simulink model "RoboPies"  (R2025b)
settings: Solver=ode23t  StartTime=0.0  StopTime=Tf  RelTol=1e-2  AbsTol=1e-2  EnableMultiTasking=on
values from neighbouring files (symbols this model uses):
  k = 2    [init_PID.m]
  x = 0.25    [init_PID.m]
undefined symbols (not defined in the file or in its folder): bias, foot_radius, ground_offset, hip_max_angle, hip_min_angle, initial_hip_angle, initial_knee_angle, knee_max_angle, knee_min_angle, lower_leg, max_a, max_friction_force, max_hip_speed, max_knee_speed, max_magnitude_force, max_torque, max_v, torso, upper_leg, X, Y, Z
libraries: nesl_utility x44, sm_lib x36, rllib x1
(part 1 of 2)
settings Model: Creator=filip  LastModifiedBy=filip
settings SolverCC: ZeroCrossAlgorithm=Adaptive  MaxZcPerStep=1.0
settings DataIOCC: LimitDataPoints=on  MaxDataPoints=10000
settings OptimizationCC: ReuseModelBlockBuffer=off  LifeSpan=inf
settings DebuggingCC: AlgebraicLoopMsg=none  UnconnectedInputMsg=warning  UnconnectedOutputMsg=warning  UnconnectedLineMsg=warning  AllowSymbolicDim=off  SubsystemReferenceDiagnosticForUnitTest=warning  SFUnexpectedBacktrackingDiag=warning  SFNoUnconditionalDefaultTransitionDiag=warning  SFExecutionAtInitializationDiag=none  ArithmeticOperatorsInVariantConditions=warning
settings ModelReferenceCC: EnableRefExpFcnMdlSchedulingChecks=on
settings SFSimCC: SimUseLocalCustomCode=off  CustomCodeUndefinedFunction=UseInterfaceOnly
settings RTWCC: RTWUseLocalCustomCode=off  GPUComputeCapability=3.5  DLArmComputeVersion=19.05
settings CodeAppCC: StateflowObjectComments=on
settings GRTTargetCC: TargetLangStandard=C89/C90 (ANSI)
settings ConfigComp: CovMetricSettings=dw  CovSaveCumulativeToWorkspaceVar=on  CovSaveSingleToWorkspaceVar=on  CovExternalEMLEnable=off  CovSFcnEnable=off
settings SimscapeCC: SimscapeLogType=all  SimscapeLogSimulationStatistics=on  SimscapeLogDataHistory=10000.0

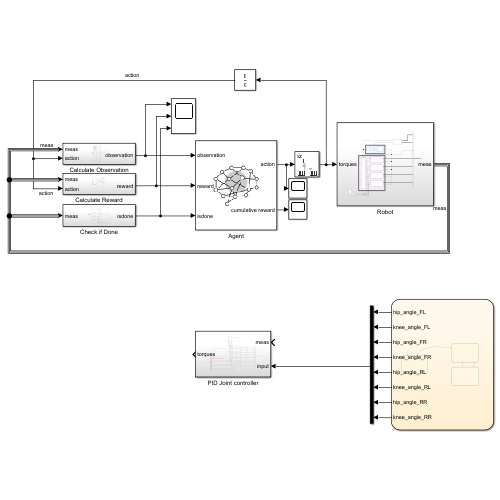
[thumbnail: Simulink's stored preview of the top-level diagram]
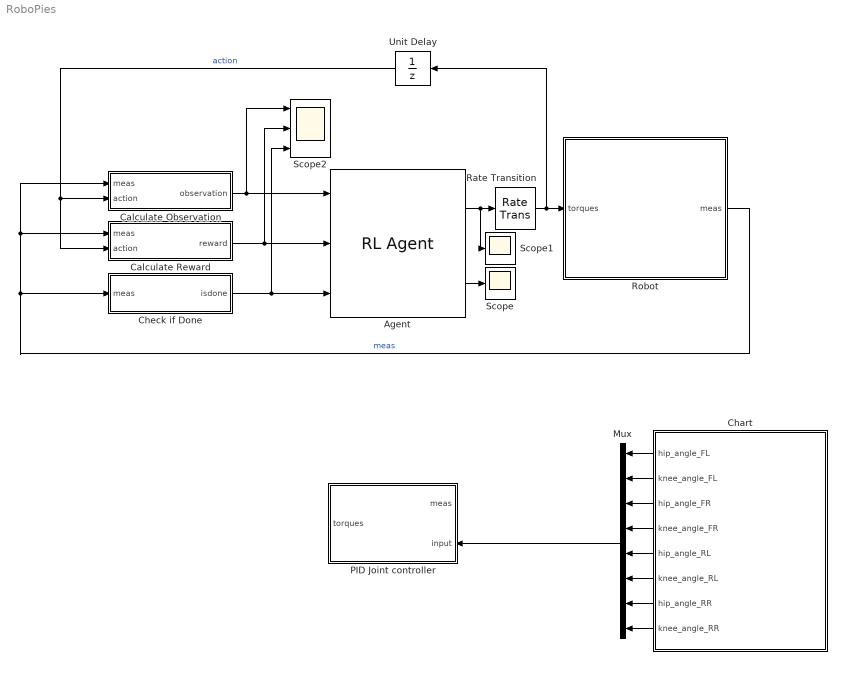
== system RoboPies ==
  Agent : rllib/RL Agent  Agent=agent  ExternalActionAsInput=off  ProvideLastAction=off  ProvideCumRwd=on  TreatAsDirectFeedthrough=on  UseStrictObservationDataTypes=off
  Calculate Observation : Subsystem
  Calculate Reward : Subsystem
  Chart : Stateflow chart  TreatAsAtomicUnit=on
  Check if Done : Subsystem
  Mux : Mux  Inputs=8
  PID Joint controller : Subsystem
  Rate Transition : RateTransition
  Robot : Subsystem
  Scope : Scope
  Scope1 : Scope
      settings: ActiveDisplayYMinimum=-2.81408298770246  ActiveDisplayYMaximum=3.6973431282332014  DataLoggingVariableName=ScopeData2
  Scope2 : Scope  NumInputPorts=3
      settings: ActiveDisplayYMinimum=-11.968223752166544  ActiveDisplayYMaximum=10.451088168830223  DataLoggingVariableName=ScopeData4
  Unit Delay : UnitDelay  SampleTime=-1  HasFrameUpgradeWarning=on
  wires:
  Chart/3(hip_angle_FR) -> Mux/3
  Chart/5(hip_angle_RL) -> Mux/5
  Chart/7(hip_angle_RR) -> Mux/7
  Chart/1(hip_angle_FL) -> Mux/1
  Chart/6(knee_angle_RL) -> Mux/6
  Chart/2(knee_angle_FL) -> Mux/2
  Chart/4(knee_angle_FR) -> Mux/4
  Chart/8(knee_angle_RR) -> Mux/8
  Mux/1 -> PID Joint controller/2(input)
  Calculate Reward/1(reward) -> Scope2/2, Agent/2
  Calculate Observation/1(observation) -> Scope2/1, Agent/1
  Robot/1(meas) -> Calculate Observation/1(meas), Calculate Reward/1(meas), Check if Done/1(meas)  "meas"
  Unit Delay/1 -> Calculate Reward/2(action), Calculate Observation/2(action)  "action"
  Check if Done/1(isdone) -> Scope2/3, Agent/3
  Agent/2 -> Scope/1
  Agent/1 -> Rate Transition/1, Scope1/1
  Rate Transition/1 -> Robot/1(torques), Unit Delay/1

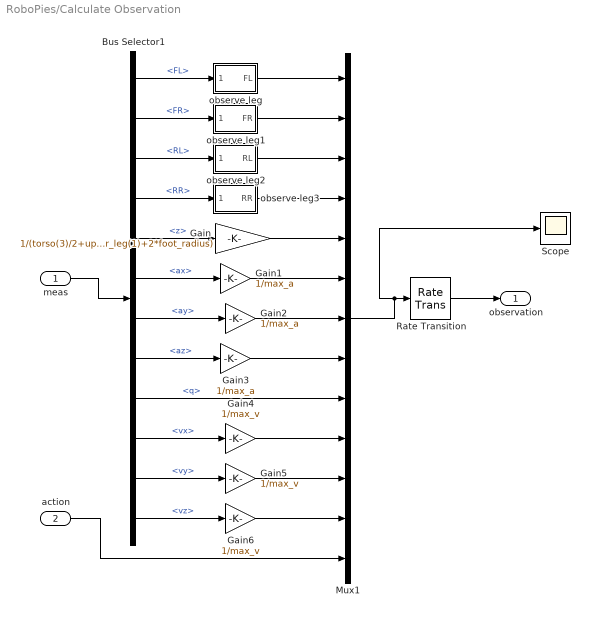
== system RoboPies/Calculate Observation ==
  meas : Inport
  action : Inport  Port=2
  Bus Selector1 : BusSelector  OutputSignals=FL,FR,RL,RR,translation.z,translation.ax,translation.ay,translation.az,rotation.q,translation.vx,translation.vy,translation.vz
  Gain : Gain  Gain=1/(torso(3)/2+upper_leg(1)+lower_leg(1)+2*foot_radius)
  Gain1 : Gain  Gain=1/max_a
  Gain2 : Gain  Gain=1/max_a
  Gain3 : Gain  Gain=1/max_a
  Gain4 : Gain  Gain=1/max_v
  Gain5 : Gain  Gain=1/max_v
  Gain6 : Gain  Gain=1/max_v
  Mux1 : Mux  Inputs=13
  Rate Transition : RateTransition  OutPortSampleTime=T
  Scope : Scope
      settings: ActiveDisplayYMinimum=-5.1137479560715171  ActiveDisplayYMaximum=2.9584463962824925  DataLoggingVariableName=ScopeData10
  observe leg : Subsystem
  observe leg1 : Subsystem
  observe leg2 : Subsystem
  observe leg3 : Subsystem
  observation : Outport
  wires:
  meas/1 -> Bus Selector1/1
  Rate Transition/1 -> observation/1
  Mux1/1 -> Scope/1, Rate Transition/1
  Bus Selector1/1 -> observe leg/1(<FL>)  "<FL>"
  Bus Selector1/2 -> observe leg1/1(<FR>)  "<FR>"
  Bus Selector1/3 -> observe leg2/1(<RL>)  "<RL>"
  Bus Selector1/4 -> observe leg3/1(<RR>)  "<RR>"
  observe leg3/1(RR) -> Mux1/4
  observe leg2/1(RL) -> Mux1/3
  observe leg1/1(FR) -> Mux1/2
  Bus Selector1/5 -> Gain/1  "<z>"
  Gain/1 -> Mux1/5
  Bus Selector1/6 -> Gain1/1  "<ax>"
  Bus Selector1/8 -> Gain3/1  "<az>"
  Bus Selector1/7 -> Gain2/1  "<ay>"
  Gain1/1 -> Mux1/6
  Gain2/1 -> Mux1/7
  Gain3/1 -> Mux1/8
  observe leg/1(FL) -> Mux1/1
  Bus Selector1/9 -> Mux1/9  "<q>"
  action/1 -> Mux1/13
  Bus Selector1/10 -> Gain4/1  "<vx>"
  Gain4/1 -> Mux1/10
  Gain5/1 -> Mux1/11
  Bus Selector1/11 -> Gain5/1  "<vy>"
  Bus Selector1/12 -> Gain6/1  "<vz>"
  Gain6/1 -> Mux1/12

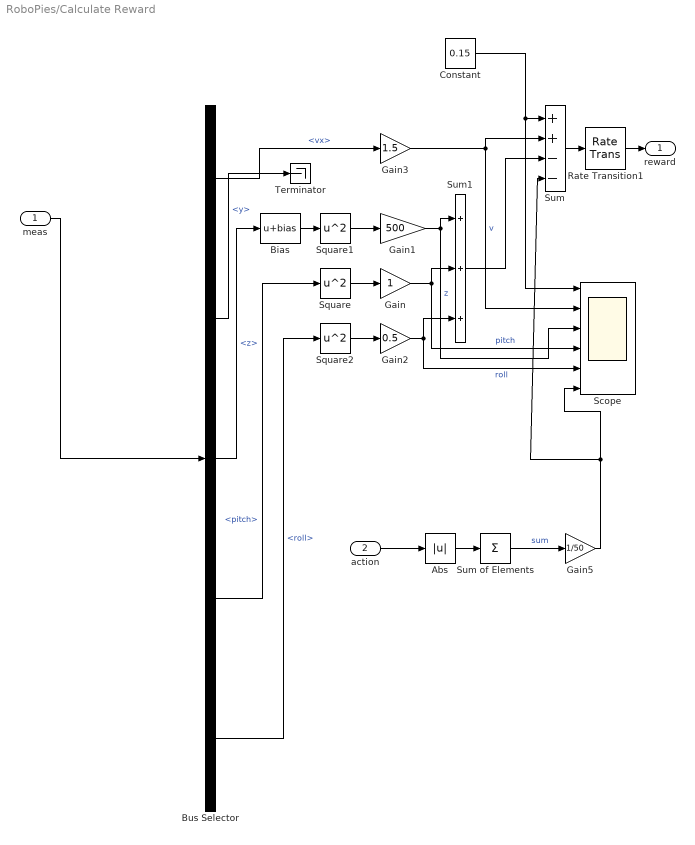
== system RoboPies/Calculate Reward ==
  meas : Inport
  action : Inport  Port=2
  Abs : Abs  SaturateOnIntegerOverflow=off
  Bias : Bias  Bias=bias  SaturateOnIntegerOverflow=off
  Bus Selector : BusSelector  OutputSignals=translation.vx,translation.y,translation.z,rotation.pitch,rotation.roll
  Constant : Constant  Value=0.15
  Gain : Gain
  Gain1 : Gain  Gain=500
  Gain2 : Gain  Gain=0.5
  Gain3 : Gain  Gain=1.5
  Gain5 : Gain  Gain=1/50
  Rate Transition1 : RateTransition  OutPortSampleTime=T
  Scope : Scope  NumInputPorts=6
      settings: ActiveDisplayYMinimum=-0.48373774424598659  ActiveDisplayYMaximum=0.73158023677854034  DataLoggingVariableName=ScopeData7
  Square : Math  Operator=square
  Square1 : Math  Operator=square
  Square2 : Math  Operator=square
  Sum : Sum  Inputs=++--
  Sum of Elements : Sum  Inputs=+
  Sum1 : Sum  Inputs=+++
  Terminator : Terminator
  reward : Outport
  wires:
  meas/1 -> Bus Selector/1
  Bus Selector/3 -> Bias/1  "<z>"
  Bias/1 -> Square1/1
  Square1/1 -> Gain1/1
  Bus Selector/2 -> Terminator/1  "<y>"
  Square/1 -> Gain/1
  Square2/1 -> Gain2/1
  Gain1/1 -> Sum1/1, Scope/3  "z"
  Gain/1 -> Sum1/2, Scope/4  "pitch"
  Gain2/1 -> Sum1/3, Scope/5  "roll"
  Bus Selector/4 -> Square/1  "<pitch>"
  Bus Selector/5 -> Square2/1  "<roll>"
  Sum1/1 -> Sum/3
  Gain3/1 -> Sum/2, Scope/2  "v"
  Constant/1 -> Scope/1, Sum/1
  Sum/1 -> Rate Transition1/1
  Bus Selector/1 -> Gain3/1  "<vx>"
  Sum of Elements/1 -> Gain5/1  "sum"
  Gain5/1 -> Sum/4, Scope/6
  Rate Transition1/1 -> reward/1
  action/1 -> Abs/1
  Abs/1 -> Sum of Elements/1

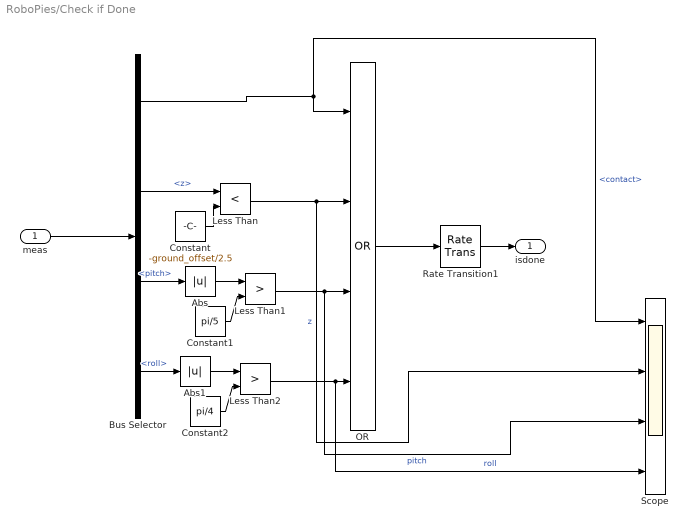
== system RoboPies/Check if Done ==
  meas : Inport
  Abs : Abs  SaturateOnIntegerOverflow=off
  Abs1 : Abs  SaturateOnIntegerOverflow=off
  Bus Selector : BusSelector  OutputSignals=contact,translation.z,rotation.pitch,rotation.roll
  Constant : Constant  Value=-ground_offset/2.5
  Constant1 : Constant  Value=pi/5
  Constant2 : Constant  Value=pi/4
  Less Than : RelationalOperator  Operator=<  OutDataTypeStr=boolean  RndMeth=Simplest  InputSameDT=off
  Less Than1 : RelationalOperator  Operator=>  OutDataTypeStr=boolean  RndMeth=Simplest  InputSameDT=off
  Less Than2 : RelationalOperator  Operator=>  OutDataTypeStr=boolean  RndMeth=Simplest  InputSameDT=off
  OR : Logic  Operator=OR  Inputs=4  AllPortsSameDT=off  OutDataTypeStr=boolean
  Rate Transition1 : RateTransition  OutPortSampleTime=T
  Scope : Scope  NumInputPorts=4
      settings: ActiveDisplayYMinimum=-0.11300019592408958  ActiveDisplayYMaximum=1.1369998040759106  DataLoggingVariableName=ScopeData9
  isdone : Outport
  wires:
  meas/1 -> Bus Selector/1
  Bus Selector/1 -> OR/1, Scope/1  "<contact>"
  OR/1 -> Rate Transition1/1
  Rate Transition1/1 -> isdone/1
  Bus Selector/2 -> Less Than/1  "<z>"
  Constant/1 -> Less Than/2
  Less Than/1 -> OR/2, Scope/2  "z"
  Bus Selector/3 -> Abs/1  "<pitch>"
  Abs/1 -> Less Than1/1
  Constant1/1 -> Less Than1/2
  Less Than1/1 -> Scope/3, OR/3  "pitch"
  Less Than2/1 -> Scope/4, OR/4  "roll"
  Bus Selector/4 -> Abs1/1  "<roll>"
  Abs1/1 -> Less Than2/1
  Constant2/1 -> Less Than2/2

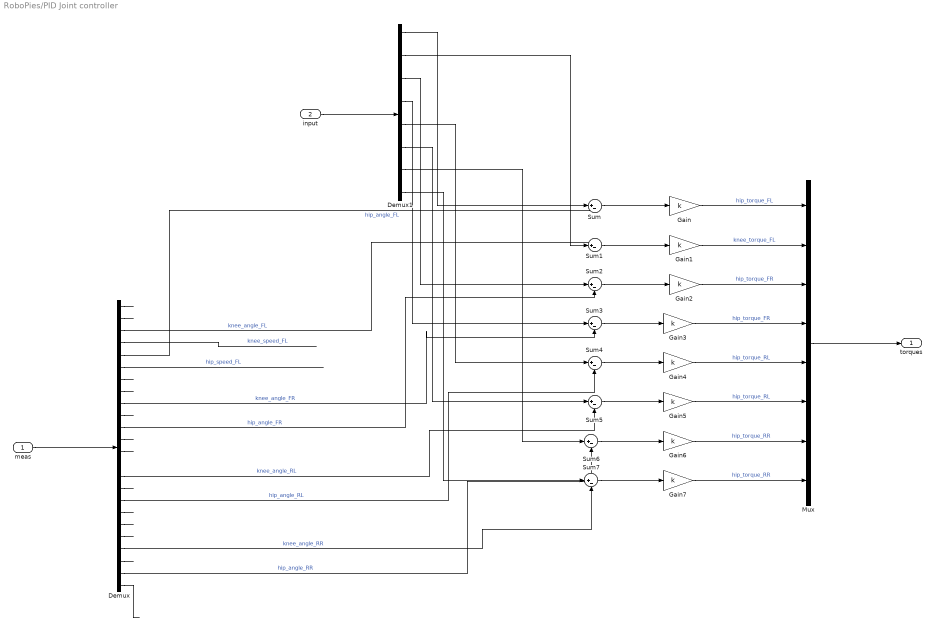
== system RoboPies/PID Joint controller ==
  meas : Inport
  input : Inport  Port=2
  Demux : Demux  Outputs=24
  Demux1 : Demux  Outputs=8
  Gain{,1..7} (8 alike) : Gain  Gain=k
  Mux : Mux  Inputs=8
  Sum{,1..7} (8 alike) : Sum  Inputs=|+-
  torques : Outport
  wires:
  Demux/5 -> Sum/2  "hip_angle_FL"
  Sum2/1 -> Gain2/1
  Gain4/1 -> Mux/5  "hip_torque_RL"
  Demux/1 -> ?
  Demux1/1 -> Sum/1
  Demux/21 -> Sum7/2  "knee_angle_RR"
  Gain3/1 -> Mux/4  "hip_torque_FR"
  Sum/1 -> Gain/1
  Demux/3 -> Sum1/2  "knee_angle_FL"
  Gain1/1 -> Mux/2  "knee_torque_FL"
  Gain2/1 -> Mux/3  "hip_torque_FR"
  Demux/6 -> ?  "hip_speed_FL"
  Gain5/1 -> Mux/6  "hip_torque_RL"
  Demux/7 -> ?
  Sum3/1 -> Gain3/1
  Demux/9 -> Sum3/2  "knee_angle_FR"
  Gain/1 -> Mux/1  "hip_torque_FL"
  Demux1/2 -> Sum1/1
  Sum1/1 -> Gain1/1
  Demux/16 -> ?
  Sum7/1 -> Gain7/1
  Demux/13 -> ?
  Demux1/3 -> Sum2/1
  Demux/8 -> ?
  Demux1/4 -> Sum3/1
  Sum4/1 -> Gain4/1
  Sum5/1 -> Gain5/1
  Demux/23 -> Sum6/2  "hip_angle_RR"
  Demux/19 -> ?
  Gain6/1 -> Mux/7  "hip_torque_RR"
  Sum6/1 -> Gain6/1
  Demux/18 -> ?
  Demux/11 -> Sum2/2  "hip_angle_FR"
  Gain7/1 -> Mux/8  "hip_torque_RR"
  Mux/1 -> torques/1
  meas/1 -> Demux/1
  Demux/10 -> ?
  Demux/2 -> ?
  Demux/12 -> ?
  Demux/15 -> Sum5/2  "knee_angle_RL"
  Demux/17 -> Sum4/2  "hip_angle_RL"
  Demux/22 -> ?
  Demux/20 -> ?
  Demux/24 -> ?
  Demux/4 -> ?  "knee_speed_FL"
  Demux1/5 -> Sum4/1
  Demux1/6 -> Sum5/1
  Demux1/7 -> Sum6/1
  Demux1/8 -> Sum7/1
  input/1 -> Demux1/1

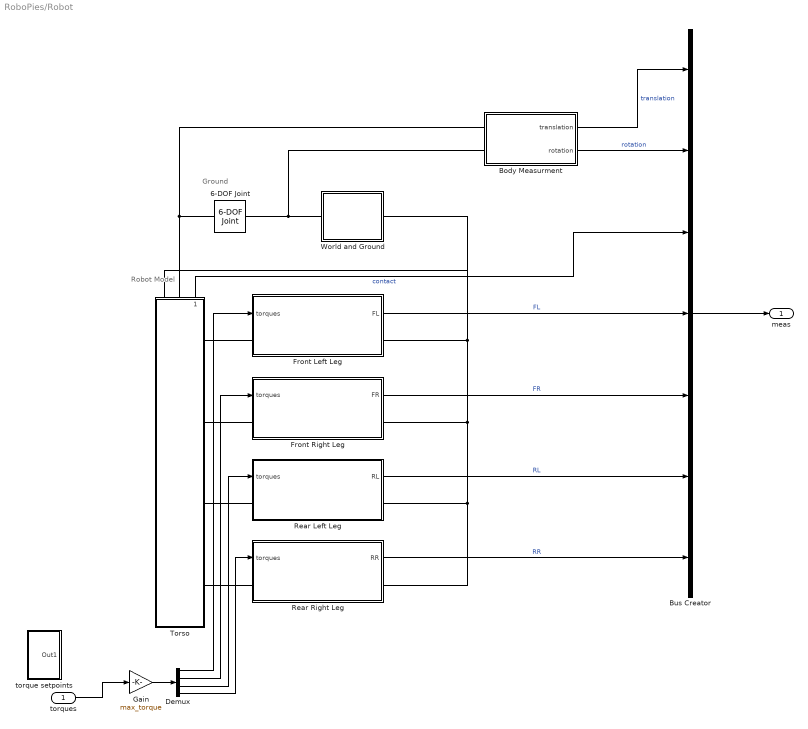
== system RoboPies/Robot ==
  note: Robot Model
  note: Ground
  torques : Inport
  6-DOF Joint : sm_lib/Joints/6-DOF Joint  JointMode=Normal  CompositeWrenchDir=FollowerOnBase  CompositeWrenchFrame=BaseFrame  SenseConstraintForce=off  SenseConstraintTorque=off  SenseTotalForce=off  SenseTotalTorque=off  PxPositionTargetSpecify=off  PxPositionTargetPriority=High  PxPositionTargetValue=0  PxPositionTargetValueUnits=m  PxVelocityTargetSpecify=off  PxVelocityTargetPriority=High  PxVelocityTargetValue=0  PxVelocityTargetValueUnits=m/s  PxEquilibriumPosition=0  PxEquilibriumPositionUnits=m  PxSpringStiffness=0  PxSpringStiffnessUnits=N/m  PxDampingCoefficient=0  PxDampingCoefficientUnits=N/(m/s)  PxLowerLimitSpecify=off  PxLowerLimitBound=-1  PxLowerLimitBoundUnits=m  PxLowerLimitStiffness=1e6  PxLowerLimitStiffnessUnits=N/m  PxLowerLimitDamping=1e3  PxLowerLimitDampingUnits=N/(m/s)  PxLowerLimitTransitionRegionWidth=1e-4  PxLowerLimitTransitionRegionWidthUnits=m  PxUpperLimitSpecify=off  PxUpperLimitBound=1  PxUpperLimitBoundUnits=m  PxUpperLimitStiffness=1e6  PxUpperLimitStiffnessUnits=N/m  PxUpperLimitDamping=1e3  PxUpperLimitDampingUnits=N/(m/s)  PxUpperLimitTransitionRegionWidth=1e-4  PxUpperLimitTransitionRegionWidthUnits=m  PxTorqueActuationMode=NoTorque  PxMotionActuationMode=ComputedMotion  PxSensePosition=off  PxSenseVelocity=off  PxSenseAcceleration=off  PxSenseTorqueForce=off  PxSenseLowerLimitTorqueForce=off  PxSenseUpperLimitTorqueForce=off  PyPositionTargetSpecify=off  PyPositionTargetPriority=High  PyPositionTargetValue=0  PyPositionTargetValueUnits=m  PyVelocityTargetSpecify=off  PyVelocityTargetPriority=High  PyVelocityTargetValue=0  PyVelocityTargetValueUnits=m/s  PyEquilibriumPosition=0  PyEquilibriumPositionUnits=m  PySpringStiffness=0  PySpringStiffnessUnits=N/m  PyDampingCoefficient=0  PyDampingCoefficientUnits=N/(m/s)  PyLowerLimitSpecify=off  PyLowerLimitBound=-1  PyLowerLimitBoundUnits=m  PyLowerLimitStiffness=1e6  PyLowerLimitStiffnessUnits=N/m  PyLowerLimitDamping=1e3  PyLowerLimitDampingUnits=N/(m/s)  PyLowerLimitTransitionRegionWidth=1e-4  PyLowerLimitTransitionRegionWidthUnits=m  PyUpperLimitSpecify=off  PyUpperLimitBound=1  PyUpperLimitBoundUnits=m  PyUpperLimitStiffness=1e6  PyUpperLimitStiffnessUnits=N/m  PyUpperLimitDamping=1e3  PyUpperLimitDampingUnits=N/(m/s)  PyUpperLimitTransitionRegionWidth=1e-4  PyUpperLimitTransitionRegionWidthUnits=m  PyTorqueActuationMode=NoTorque  PyMotionActuationMode=ComputedMotion  PySensePosition=off  PySenseVelocity=off  PySenseAcceleration=off  PySenseTorqueForce=off  PySenseLowerLimitTorqueForce=off  PySenseUpperLimitTorqueForce=off  PzPositionTargetSpecify=off  PzPositionTargetPriority=High  PzPositionTargetValue=0  PzPositionTargetValueUnits=m  PzVelocityTargetSpecify=off  PzVelocityTargetPriority=High  PzVelocityTargetValue=0  PzVelocityTargetValueUnits=m/s  PzEquilibriumPosition=0  PzEquilibriumPositionUnits=m  PzSpringStiffness=0  PzSpringStiffnessUnits=N/m  PzDampingCoefficient=0  PzDampingCoefficientUnits=N/(m/s)  PzLowerLimitSpecify=off  PzLowerLimitBound=-1  PzLowerLimitBoundUnits=m  PzLowerLimitStiffness=1e6  PzLowerLimitStiffnessUnits=N/m  PzLowerLimitDamping=1e3  PzLowerLimitDampingUnits=N/(m/s)  PzLowerLimitTransitionRegionWidth=1e-4  PzLowerLimitTransitionRegionWidthUnits=m  PzUpperLimitSpecify=off  PzUpperLimitBound=1  PzUpperLimitBoundUnits=m  PzUpperLimitStiffness=1e6  PzUpperLimitStiffnessUnits=N/m  PzUpperLimitDamping=1e3  PzUpperLimitDampingUnits=N/(m/s)  PzUpperLimitTransitionRegionWidth=1e-4  PzUpperLimitTransitionRegionWidthUnits=m  PzTorqueActuationMode=NoTorque  PzMotionActuationMode=ComputedMotion  PzSensePosition=off  PzSenseVelocity=off  PzSenseAcceleration=off  PzSenseTorqueForce=off  PzSenseLowerLimitTorqueForce=off  PzSenseUpperLimitTorqueForce=off  SphPositionTargetSpecify=off  SphPositionTargetPriority=High  SphPositionTargetRotationMethod=None  SphPositionTargetFollAlignAxisA=+X  SphPositionTargetBaseAlignAxisA=+Y  SphPositionTargetFollAlignAxisB=+Y  SphPositionTargetBaseAlignAxisB=+Z  SphPositionTargetRotationStandardAxis=+Z  SphPositionTargetRotationAngle=0  SphPositionTargetRotationAngleUnits=deg  SphPositionTargetRotationArbitraryAxis=[0 0 1]  SphPositionTargetRotationSequenceAxes=FollowerAxes  SphPositionTargetRotationSequence=XYX  SphPositionTargetRotationSequenceAngles=[0 0 0]  SphPositionTargetRotationSequenceAnglesUnits=deg  SphPositionTargetRotationMatrix=[1 0 0;0 1 0;0 0 1]  SphPositionTargetQuaternion=[1 0 0 0]  SphVelocityTargetSpecify=off  SphVelocityTargetPriority=High  SphVelocityTargetValue=[0 0 0]  SphVelocityTargetValueUnits=deg/s  SphVelocityTargetInFollowerFrame=on  SphEqPosRotationMethod=None  SphEqPosFollAlignAxisA=+X  SphEqPosBaseAlignAxisA=+Y  SphEqPosFollAlignAxisB=+Y  SphEqPosBaseAlignAxisB=+Z  SphEqPosRotationStandardAxis=+Z  SphEqPosRotationAngle=0  SphEqPosRotationAngleUnits=deg  SphEqPosRotationArbitraryAxis=[0 0 1]  SphEqPosRotationSequenceAxes=FollowerAxes  SphEqPosRotationSequence=XYX  SphEqPosRotationSequenceAngles=[0 0 0]  SphEqPosRotationSequenceAnglesUnits=deg  SphEqPosRotationMatrix=[1 0 0;0 1 0;0 0 1]  SphEqPosQuaternion=[1 0 0 0]  SphSpringStiffness=0  SphSpringStiffnessUnits=N*m/deg  SphDampingCoefficient=0  SphDampingCoefficientUnits=N*m/(deg/s)  SphLowerLimitSpecify=off  SphLowerLimitBound=15  SphLowerLimitBoundUnits=deg  SphLowerLimitStiffness=1e4  SphLowerLimitStiffnessUnits=N*m/deg  SphLowerLimitDamping=10  SphLowerLimitDampingUnits=N*m/(deg/s)  SphLowerLimitTransitionRegionWidth=0.1  SphLowerLimitTransitionRegionWidthUnits=deg  SphUpperLimitSpecify=off  SphUpperLimitBound=45  SphUpperLimitBoundUnits=deg  SphUpperLimitStiffness=1e4  SphUpperLimitStiffnessUnits=N*m/deg  SphUpperLimitDamping=10  SphUpperLimitDampingUnits=N*m/(deg/s)  SphUpperLimitTransitionRegionWidth=0.1  SphUpperLimitTransitionRegionWidthUnits=deg  SphTorqueActuationMode=NoTorque  SphActuateTorqueX=off  SphActuateTorqueY=off  SphActuateTorqueZ=off  SphActuateTorque=off  SphActuationFrame=BaseFrame  SphSensePosition=off  SphSenseVelocityX=off  SphSenseVelocityY=off  SphSenseVelocityZ=off  SphSenseVelocity=off  SphSenseAccelerationX=off  SphSenseAccelerationY=off  SphSenseAccelerationZ=off  SphSenseAcceleration=off  SphSenseLowerLimitTorqueMag=off  SphSenseUpperLimitTorqueMag=off  SphSensingFrame=BaseFrame
  Body Measurment : Subsystem
  Bus Creator : BusCreator  Inputs=7
  Demux : Demux
  Front Left Leg : Subsystem
      settings: PortSchema="{\"entries\":[{\"content\":{\"sides\":[{\"content\":{\"connectorIds\":[\"LConn1\",\"In1\"]},\"type\":\"ConnectorPlacement.EquallySpacedRectSide\",\"uuid\":\"67cc346d-8093-4a90-beea-ad102c28a529\"},{\"content\":{\"connectorIds\":[\"RConn1\",\"Out1\"],\"side\":\"RIGHT\"},\"type\":\"ConnectorPlacement.EquallySpacedRectSide\",\"uuid\":\"a41fbdac-a3bc-454a-9a02-c1548b06e168\"},{\"content\":{\"side\":\"TOP\"},\"type\":\"ConnectorPlacement.EquallySpacedRectSide\",\"uuid\":\"2db3de25-17b9-42a2-b258-04f424c8657a\"}]},\"type\":\"ConnectorPlacement.EquallySpacedConnector\",\"uuid\":\"8d839d8f-2b1b-4b58-b696-304cf56daaed\"}],\"packageUris\":[\"http://schema.mathworks.com/mf0/Connector/R2020b\"],\"version\":\"1.0\"}"
  Front Right Leg : Subsystem
      settings: PortSchema="{\"entries\":[{\"content\":{\"sides\":[{\"content\":{\"connectorIds\":[\"LConn1\",\"In1\"]},\"type\":\"ConnectorPlacement.EquallySpacedRectSide\",\"uuid\":\"34c80378-d001-4ef7-8c50-56da40a680d3\"},{\"content\":{\"connectorIds\":[\"RConn1\",\"Out1\"],\"side\":\"RIGHT\"},\"type\":\"ConnectorPlacement.EquallySpacedRectSide\",\"uuid\":\"d8c47c46-5f9d-4ebc-b52e-d8bb210754e6\"},{\"content\":{\"side\":\"TOP\"},\"type\":\"ConnectorPlacement.EquallySpacedRectSide\",\"uuid\":\"9923bc19-0faa-4da1-9dcb-df221e5d47f7\"}]},\"type\":\"ConnectorPlacement.EquallySpacedConnector\",\"uuid\":\"13843bdb-d0bb-4acc-95de-2d753d5922a7\"}],\"packageUris\":[\"http://schema.mathworks.com/mf0/Connector/R2020b\"],\"version\":\"1.0\"}"
  Gain : Gain  Gain=max_torque
  Rear Left Leg : Subsystem
      settings: PortSchema="{\"entries\":[{\"content\":{\"sides\":[{\"content\":{\"connectorIds\":[\"LConn1\",\"In1\"]},\"type\":\"ConnectorPlacement.EquallySpacedRectSide\",\"uuid\":\"34c80378-d001-4ef7-8c50-56da40a680d3\"},{\"content\":{\"connectorIds\":[\"RConn1\",\"Out1\"],\"side\":\"RIGHT\"},\"type\":\"ConnectorPlacement.EquallySpacedRectSide\",\"uuid\":\"d8c47c46-5f9d-4ebc-b52e-d8bb210754e6\"},{\"content\":{\"side\":\"TOP\"},\"type\":\"ConnectorPlacement.EquallySpacedRectSide\",\"uuid\":\"9923bc19-0faa-4da1-9dcb-df221e5d47f7\"}]},\"type\":\"ConnectorPlacement.EquallySpacedConnector\",\"uuid\":\"13843bdb-d0bb-4acc-95de-2d753d5922a7\"}],\"packageUris\":[\"http://schema.mathworks.com/mf0/Connector/R2020b\"],\"version\":\"1.0\"}"
  Rear Right Leg : Subsystem
      settings: PortSchema="{\"entries\":[{\"content\":{\"sides\":[{\"content\":{\"connectorIds\":[\"LConn1\",\"In1\"]},\"type\":\"ConnectorPlacement.EquallySpacedRectSide\",\"uuid\":\"34c80378-d001-4ef7-8c50-56da40a680d3\"},{\"content\":{\"connectorIds\":[\"RConn1\",\"Out1\"],\"side\":\"RIGHT\"},\"type\":\"ConnectorPlacement.EquallySpacedRectSide\",\"uuid\":\"d8c47c46-5f9d-4ebc-b52e-d8bb210754e6\"},{\"content\":{\"side\":\"TOP\"},\"type\":\"ConnectorPlacement.EquallySpacedRectSide\",\"uuid\":\"9923bc19-0faa-4da1-9dcb-df221e5d47f7\"}]},\"type\":\"ConnectorPlacement.EquallySpacedConnector\",\"uuid\":\"13843bdb-d0bb-4acc-95de-2d753d5922a7\"}],\"packageUris\":[\"http://schema.mathworks.com/mf0/Connector/R2020b\"],\"version\":\"1.0\"}"
  Torso : Subsystem
      settings: PortSchema="{\"entries\":[{\"content\":{\"sides\":[{\"content\":{\"connectorIds\":[\"LConn1\",\"LConn2\",\"LConn3\",\"LConn4\"]},\"type\":\"ConnectorPlacement.EquallySpacedRectSide\",\"uuid\":\"8c53a05f-c94a-44be-b209-a034cec6561e\"},{\"content\":{\"side\":\"RIGHT\"},\"type\":\"ConnectorPlacement.EquallySpacedRectSide\",\"uuid\":\"a3c22973-bf74-4661-9744-7bfaa32719ac\"},{\"content\":{\"connectorIds\":[\"Out1\",\"LConn5\",\"LConn6\"],\"side\":\"TOP\"},\"type\":\"ConnectorPlacement.EquallySpacedRectSide\",\"uuid\":\"da2dd510-6694-4077-b588-65723e1f355d\"}]},\"type\":\"ConnectorPlacement.EquallySpacedConnector\",\"uuid\":\"e4e4bf1c-8f02-4a77-9d3b-bb8def7996fd\"}],\"packageUris\":[\"http://schema.mathworks.com/mf0/Connector/R2020b\"],\"version\":\"1.0\"}"
  World and Ground : Subsystem
  torque setpoints : Subsystem
  meas : Outport
  wires:
  Demux/2 -> Front Right Leg/1(torques)
  Demux/3 -> Rear Left Leg/1(torques)
  Demux/4 -> Rear Right Leg/1(torques)
  Demux/1 -> Front Left Leg/1(torques)
  Front Left Leg/1(FL) -> Bus Creator/4  "FL"
  Bus Creator/1 -> meas/1
  Front Right Leg/1(FR) -> Bus Creator/5  "FR"
  Rear Left Leg/1(RL) -> Bus Creator/6  "RL"
  Rear Right Leg/1(RR) -> Bus Creator/7  "RR"
  Torso/1(contact) -> Bus Creator/3  "contact"
  Body Measurment/2(rotation) -> Bus Creator/2  "rotation"
  Body Measurment/1(translation) -> Bus Creator/1  "translation"
  Gain/1 -> Demux/1
  torques/1 -> Gain/1
  connections:
  Front Left Leg/RConn1 -- World and Ground/LConn1 -- Torso/LConn6 -- Front Right Leg/RConn1 -- Rear Right Leg/RConn1 -- Rear Left Leg/RConn1
  Rear Right Leg/LConn1 -- Torso/LConn4
  Body Measurment/LConn2 -- 6-DOF Joint/LConn1 -- World and Ground/RConn1
  Front Right Leg/LConn1 -- Torso/LConn2
  6-DOF Joint/RConn1 -- Body Measurment/LConn1 -- Torso/LConn5
  Torso/LConn1 -- Front Left Leg/LConn1
  Rear Left Leg/LConn1 -- Torso/LConn3

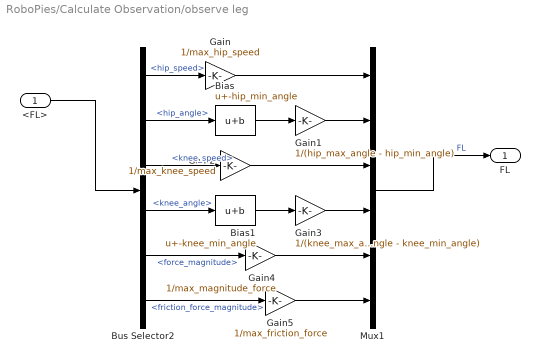
== system RoboPies/Calculate Observation/observe leg ==
  <FL> : Inport
  Bias : Bias  Bias=-hip_min_angle  SaturateOnIntegerOverflow=off
  Bias1 : Bias  Bias=-knee_min_angle  SaturateOnIntegerOverflow=off
  Bus Selector2 : BusSelector  OutputSignals=hip_speed,hip_angle,knee_speed,knee_angle,force_magnitude,friction_force_magnitude
  Gain : Gain  Gain=1/max_hip_speed
  Gain1 : Gain  Gain=1/(hip_max_angle - hip_min_angle)
  Gain2 : Gain  Gain=1/max_knee_speed
  Gain3 : Gain  Gain=1/(knee_max_angle - knee_min_angle)
  Gain4 : Gain  Gain=1/max_magnitude_force
  Gain5 : Gain  Gain=1/max_friction_force
  Mux1 : Mux  Inputs=6
  FL : Outport
  wires:
  Gain/1 -> Mux1/1
  Gain1/1 -> Mux1/2
  Bus Selector2/6 -> Gain5/1  "<friction_force_magnitude>"
  Bus Selector2/4 -> Bias1/1  "<knee_angle>"
  Bus Selector2/5 -> Gain4/1  "<force_magnitude>"
  Gain2/1 -> Mux1/3
  Gain3/1 -> Mux1/4
  Gain4/1 -> Mux1/5
  Bus Selector2/2 -> Bias/1  "<hip_angle>"
  Mux1/1 -> FL/1  "FL"
  Bias/1 -> Gain1/1
  Bus Selector2/3 -> Gain2/1  "<knee_speed>"
  Gain5/1 -> Mux1/6
  Bias1/1 -> Gain3/1
  <FL>/1 -> Bus Selector2/1
  Bus Selector2/1 -> Gain/1  "<hip_speed>"

== system RoboPies/Calculate Observation/observe leg1 ==
  <FR> : Inport
  Bias : Bias  Bias=-hip_min_angle  SaturateOnIntegerOverflow=off
  Bias1 : Bias  Bias=-knee_min_angle  SaturateOnIntegerOverflow=off
  Bus Selector2 : BusSelector  OutputSignals=hip_speed,hip_angle,knee_speed,knee_angle,force_magnitude,friction_force_magnitude
  Gain : Gain  Gain=1/max_hip_speed
  Gain1 : Gain  Gain=1/(hip_max_angle - hip_min_angle)
  Gain2 : Gain  Gain=1/max_knee_speed
  Gain3 : Gain  Gain=1/(knee_max_angle - knee_min_angle)
  Gain4 : Gain  Gain=1/max_magnitude_force
  Gain5 : Gain  Gain=1/max_friction_force
  Mux1 : Mux  Inputs=6
  FR : Outport
  wires:
  Gain/1 -> Mux1/1
  Gain1/1 -> Mux1/2
  Bus Selector2/6 -> Gain5/1  "<friction_force_magnitude>"
  Bus Selector2/4 -> Bias1/1  "<knee_angle>"
  Bus Selector2/5 -> Gain4/1  "<force_magnitude>"
  Gain2/1 -> Mux1/3
  Gain3/1 -> Mux1/4
  Gain4/1 -> Mux1/5
  Bus Selector2/2 -> Bias/1  "<hip_angle>"
  Mux1/1 -> FR/1  "FR"
  Bias/1 -> Gain1/1
  Bus Selector2/3 -> Gain2/1  "<knee_speed>"
  Gain5/1 -> Mux1/6
  Bias1/1 -> Gain3/1
  <FR>/1 -> Bus Selector2/1
  Bus Selector2/1 -> Gain/1  "<hip_speed>"

== system RoboPies/Calculate Observation/observe leg2 ==
  <RL> : Inport
  Bias : Bias  Bias=-hip_min_angle  SaturateOnIntegerOverflow=off
  Bias1 : Bias  Bias=-knee_min_angle  SaturateOnIntegerOverflow=off
  Bus Selector2 : BusSelector  OutputSignals=hip_speed,hip_angle,knee_speed,knee_angle,force_magnitude,friction_force_magnitude
  Gain : Gain  Gain=1/max_hip_speed
  Gain1 : Gain  Gain=1/(hip_max_angle - hip_min_angle)
  Gain2 : Gain  Gain=1/max_knee_speed
  Gain3 : Gain  Gain=1/(knee_max_angle - knee_min_angle)
  Gain4 : Gain  Gain=1/max_magnitude_force
  Gain5 : Gain  Gain=1/max_friction_force
  Mux1 : Mux  Inputs=6
  RL : Outport
  wires:
  Gain/1 -> Mux1/1
  Gain1/1 -> Mux1/2
  Bus Selector2/6 -> Gain5/1  "<friction_force_magnitude>"
  Bus Selector2/4 -> Bias1/1  "<knee_angle>"
  Bus Selector2/5 -> Gain4/1  "<force_magnitude>"
  Gain2/1 -> Mux1/3
  Gain3/1 -> Mux1/4
  Gain4/1 -> Mux1/5
  Bus Selector2/2 -> Bias/1  "<hip_angle>"
  Mux1/1 -> RL/1  "RL"
  Bias/1 -> Gain1/1
  Bus Selector2/3 -> Gain2/1  "<knee_speed>"
  Gain5/1 -> Mux1/6
  Bias1/1 -> Gain3/1
  <RL>/1 -> Bus Selector2/1
  Bus Selector2/1 -> Gain/1  "<hip_speed>"

== system RoboPies/Calculate Observation/observe leg3 ==
  <RR> : Inport
  Bias : Bias  Bias=-hip_min_angle  SaturateOnIntegerOverflow=off
  Bias1 : Bias  Bias=-knee_min_angle  SaturateOnIntegerOverflow=off
  Bus Selector2 : BusSelector  OutputSignals=hip_speed,hip_angle,knee_speed,knee_angle,force_magnitude,friction_force_magnitude
  Gain : Gain  Gain=1/max_hip_speed
  Gain1 : Gain  Gain=1/(hip_max_angle - hip_min_angle)
  Gain2 : Gain  Gain=1/max_knee_speed
  Gain3 : Gain  Gain=1/(knee_max_angle - knee_min_angle)
  Gain4 : Gain  Gain=1/max_magnitude_force
  Gain5 : Gain  Gain=1/max_friction_force
  Mux1 : Mux  Inputs=6
  RR : Outport
  wires:
  Gain/1 -> Mux1/1
  Gain1/1 -> Mux1/2
  Bus Selector2/6 -> Gain5/1  "<friction_force_magnitude>"
  Bus Selector2/4 -> Bias1/1  "<knee_angle>"
  Bus Selector2/5 -> Gain4/1  "<force_magnitude>"
  Gain2/1 -> Mux1/3
  Gain3/1 -> Mux1/4
  Gain4/1 -> Mux1/5
  Bus Selector2/2 -> Bias/1  "<hip_angle>"
  Mux1/1 -> RR/1  "RR"
  Bias/1 -> Gain1/1
  Bus Selector2/3 -> Gain2/1  "<knee_speed>"
  Gain5/1 -> Mux1/6
  Bias1/1 -> Gain3/1
  <RR>/1 -> Bus Selector2/1
  Bus Selector2/1 -> Gain/1  "<hip_speed>"

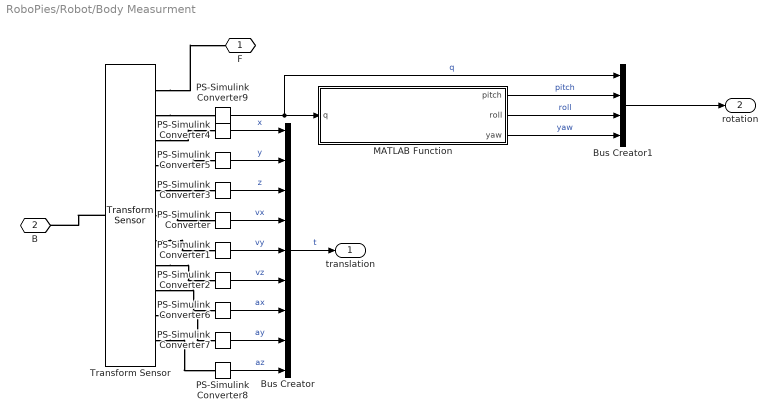
== system RoboPies/Robot/Body Measurment ==
  Bus Creator : BusCreator  Inputs=9
  Bus Creator1 : BusCreator  Inputs=4
  MATLAB Function : MATLAB Function  TreatAsAtomicUnit=on
  PS-Simulink Converter{,1..9} (10 alike) : nesl_utility/PS-Simulink Converter  PhysicalDomain=network_engine_domain  SubClassName=ps_output  LeftPortType=input  RightPortType=output  PseudoPeriodic=off  Frequencies=[]  VectorFormat=inherit  Unit=inherit  AffineConversion=off
  Transform Sensor : sm_lib/Frames and Transforms/Transform Sensor  MeasurementFrame=World  RotationSequence=XYX  SenseAngle=off  SenseAxis=off  SenseQ=on  SenseR=off  SenseRotationSequence=off  SenseOmegaX=off  SenseOmegaY=off  SenseOmegaZ=off  SenseOmega=off  SenseQDot=off  SenseRDot=off  SenseRotationSequenceDot=off  SenseAlphaX=off  SenseAlphaY=off  SenseAlphaZ=off  SenseAlpha=off  SenseQDDot=off  SenseRDDot=off  SenseX=on  SenseY=on  SenseZ=on  SenseXYZ=off  SenseRad=off  SenseAzim=off  SenseDist=off  SenseInc=off  SenseXDot=on  SenseYDot=on  SenseZDot=on  SenseXYZDot=off  SenseRadDot=off  SenseAzimDot=off  SenseDistDot=off  SenseIncDot=off  SenseXDDot=on  SenseYDDot=on  SenseZDDot=on  SenseXYZDDot=off  SenseRadDDot=off  SenseAzimDDot=off  SenseDistDDot=off  SenseIncDDot=off
  F : PMIOPort  Side=Left
  B : PMIOPort  Port=2  Side=Left
  translation : Outport
  rotation : Outport  Port=2
  wires:
  PS-Simulink Converter4/1 -> Bus Creator/1  "x"
  PS-Simulink Converter/1 -> Bus Creator/4  "vx"
  PS-Simulink Converter3/1 -> Bus Creator/3  "z"
  PS-Simulink Converter5/1 -> Bus Creator/2  "y"
  PS-Simulink Converter2/1 -> Bus Creator/6  "vz"
  PS-Simulink Converter1/1 -> Bus Creator/5  "vy"
  Bus Creator/1 -> translation/1  "t"
  PS-Simulink Converter7/1 -> Bus Creator/8  "ay"
  PS-Simulink Converter8/1 -> Bus Creator/9  "az"
  PS-Simulink Converter6/1 -> Bus Creator/7  "ax"
  PS-Simulink Converter9/1 -> Bus Creator1/1, MATLAB Function/1(q)  "q"
  Bus Creator1/1 -> rotation/1
  MATLAB Function/1(pitch) -> Bus Creator1/2  "pitch"
  MATLAB Function/2(roll) -> Bus Creator1/3  "roll"
  MATLAB Function/3(yaw) -> Bus Creator1/4  "yaw"
  connections:
  Transform Sensor/RConn6 -- PS-Simulink Converter/LConn1
  Transform Sensor/RConn7 -- PS-Simulink Converter1/LConn1
  Transform Sensor/RConn8 -- PS-Simulink Converter2/LConn1
  Transform Sensor/RConn1 -- F/RConn1
  Transform Sensor/RConn3 -- PS-Simulink Converter4/LConn1
  Transform Sensor/RConn5 -- PS-Simulink Converter3/LConn1
  Transform Sensor/RConn4 -- PS-Simulink Converter5/LConn1
  Transform Sensor/LConn1 -- B/RConn1
  Transform Sensor/RConn11 -- PS-Simulink Converter8/LConn1
  Transform Sensor/RConn9 -- PS-Simulink Converter6/LConn1
  Transform Sensor/RConn10 -- PS-Simulink Converter7/LConn1
  Transform Sensor/RConn2 -- PS-Simulink Converter9/LConn1

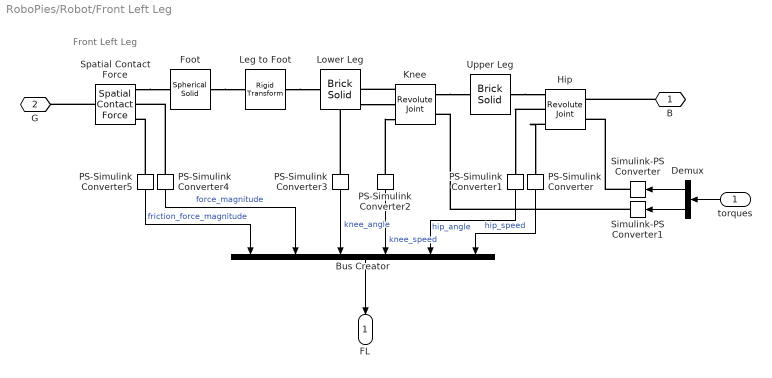
== system RoboPies/Robot/Front Left Leg ==
  note: Front Left Leg
  torques : Inport
  Bus Creator : BusCreator  Inputs=6
  Demux : Demux  Outputs=2
  Foot : sm_lib/Body Elements/Spherical Solid  SphereRadius=foot_radius  SphereRadiusUnits=m  ExportEntireGeometry=on  InertiaType=CalculateFromGeometry  BasedOnType=Density  Density=1000  DensityUnits=kg/m^3  Mass=1  MassUnits=kg  CenterOfMass=[0 0 0]  CenterOfMassUnits=m  MomentsOfInertia=[1 1 1]  MomentsOfInertiaUnits=kg*m^2  ProductsOfInertia=[0 0 0]  ProductsOfInertiaUnits=kg*m^2  GraphicType=FromGeometry  MarkerShape=Sphere  MarkerSize=10  GraphicVisPropType=SimpleVisualProperties  GraphicDiffuseColor=robot_color  GraphicOpacity=1  GraphicSpecularColor=[0.5 0.5 0.5 1.0]  GraphicAmbientColor=[0.15 0.15 0.15 1.0]  GraphicEmissiveColor=[0.0 0.0 0.0 1.0]  GraphicShininess=75  DoExposeReferenceFrame=on  SerializedFrames=<Frames/>
  Hip : sm_lib/Joints/Revolute Joint  JointMode=Normal  CompositeWrenchDir=FollowerOnBase  CompositeWrenchFrame=BaseFrame  SenseConstraintForce=off  SenseConstraintTorque=off  SenseTotalForce=off  SenseTotalTorque=off  PositionTargetSpecify=on  PositionTargetPriority=High  PositionTargetValue=initial_hip_angle  PositionTargetValueUnits=rad  VelocityTargetSpecify=off  VelocityTargetPriority=High  VelocityTargetValue=0  VelocityTargetValueUnits=deg/s  EquilibriumPosition=0  EquilibriumPositionUnits=deg  SpringStiffness=0  SpringStiffnessUnits=N*m/deg  DampingCoefficient=motor_damping  DampingCoefficientUnits=N*m*s/rad  LowerLimitSpecify=on  LowerLimitBound=hip_min_angle  LowerLimitBoundUnits=rad  LowerLimitStiffness=1e4  LowerLimitStiffnessUnits=N*m/deg  LowerLimitDamping=10  LowerLimitDampingUnits=N*m/(deg/s)  LowerLimitTransitionRegionWidth=1  LowerLimitTransitionRegionWidthUnits=deg  UpperLimitSpecify=on  UpperLimitBound=hip_max_angle  UpperLimitBoundUnits=rad  UpperLimitStiffness=1e4  UpperLimitStiffnessUnits=N*m/deg  UpperLimitDamping=10  UpperLimitDampingUnits=N*m/(deg/s)  UpperLimitTransitionRegionWidth=1  UpperLimitTransitionRegionWidthUnits=deg  TorqueActuationMode=InputTorque  MotionActuationMode=ComputedMotion  SensePosition=on  SenseVelocity=on  SenseAcceleration=off  SenseTorqueForce=off  SenseLowerLimitTorqueForce=off  SenseUpperLimitTorqueForce=off
  Knee : sm_lib/Joints/Revolute Joint  JointMode=Normal  CompositeWrenchDir=FollowerOnBase  CompositeWrenchFrame=BaseFrame  SenseConstraintForce=off  SenseConstraintTorque=off  SenseTotalForce=off  SenseTotalTorque=off  PositionTargetSpecify=on  PositionTargetPriority=High  PositionTargetValue=initial_knee_angle  PositionTargetValueUnits=rad  VelocityTargetSpecify=off  VelocityTargetPriority=High  VelocityTargetValue=0  VelocityTargetValueUnits=deg/s  EquilibriumPosition=0  EquilibriumPositionUnits=deg  SpringStiffness=0  SpringStiffnessUnits=N*m/deg  DampingCoefficient=motor_damping  DampingCoefficientUnits=N*m*s/rad  LowerLimitSpecify=on  LowerLimitBound=knee_min_angle  LowerLimitBoundUnits=rad  LowerLimitStiffness=1e4  LowerLimitStiffnessUnits=N*m/deg  LowerLimitDamping=10  LowerLimitDampingUnits=N*m/(deg/s)  LowerLimitTransitionRegionWidth=1  LowerLimitTransitionRegionWidthUnits=deg  UpperLimitSpecify=on  UpperLimitBound=knee_max_angle  UpperLimitBoundUnits=rad  UpperLimitStiffness=1e4  UpperLimitStiffnessUnits=N*m/deg  UpperLimitDamping=10  UpperLimitDampingUnits=N*m/(deg/s)  UpperLimitTransitionRegionWidth=1  UpperLimitTransitionRegionWidthUnits=deg  TorqueActuationMode=InputTorque  MotionActuationMode=ComputedMotion  SensePosition=on  SenseVelocity=on  SenseAcceleration=off  SenseTorqueForce=off  SenseLowerLimitTorqueForce=off  SenseUpperLimitTorqueForce=off
  Leg to Foot : sm_lib/Frames and Transforms/Rigid Transform  RotationMethod=None  FollAlignAxisA=+X  BaseAlignAxisA=+Y  FollAlignAxisB=+Y  BaseAlignAxisB=+Z  RotationStandardAxis=+Z  RotationAngle=0  RotationAngleUnits=deg  RotationArbitraryAxis=[0 0 1]  RotationSequenceAxes=FollowerAxes  RotationSequence=XYX  RotationSequenceAngles=[0 0 0]  RotationSequenceAnglesUnits=deg  RotationMatrix=[1 0 0;0 1 0;0 0 1]  Quaternion=[1 0 0 0]  TranslationMethod=StandardAxis  TranslationCartesianOffset=[0 0 0]  TranslationCartesianOffsetUnits=m  TranslationStandardAxis=+Z  TranslationStandardOffset=0.8*foot_radius  TranslationStandardOffsetUnits=m  TranslationROffset=0  TranslationROffsetUnits=m  TranslationThetaOffset=0  TranslationThetaOffsetUnits=deg  TranslationZOffset=0  TranslationZOffsetUnits=m
  Lower Leg : sm_lib/Body Elements/Brick Solid  BrickDimensions=lower_leg  BrickDimensionsUnits=m  ExportEntireGeometry=off  InertiaType=CalculateFromGeometry  BasedOnType=Density  Density=density  DensityUnits=kg/m^3  Mass=1  MassUnits=kg  CenterOfMass=[0 0 0]  CenterOfMassUnits=m  MomentsOfInertia=[1 1 1]  MomentsOfInertiaUnits=kg*m^2  ProductsOfInertia=[0 0 0]  ProductsOfInertiaUnits=kg*m^2  GraphicType=FromGeometry  MarkerShape=Sphere  MarkerSize=10  GraphicVisPropType=SimpleVisualProperties  GraphicDiffuseColor=robot_color  GraphicOpacity=1  GraphicSpecularColor=[0.5 0.5 0.5 1.0]  GraphicAmbientColor=[0.15 0.15 0.15 1.0]  GraphicEmissiveColor=[0.0 0.0 0.0 1.0]  GraphicShininess=75  DoExposeReferenceFrame=off  SerializedFrames=|
      | <Frames>
      | 
      |   <Frame>
      |     <Id>Frame1</Id>
      |     <Value>
      |       <Name>F1</Name>
      |       <Origin>
      |         <Source>GeometricFeature</Source>
      |         <FeatureName>-x -y curve</FeatureName>
      |       </Origin>
      |       <PrimaryAxis>
      |         <DefinedDirection>+Z</DefinedDirection>
      |         <Source>GeometricFeature</Source>
      |         <SourceDirection>+Z</SourceDirection>
      |         <FeatureName>-y surface</FeatureName>
      |       </PrimaryAxis>
      |       <SecondaryAxis>
      |         <DefinedDirection>+X</DefinedDirection>
      |         <Source>GeometricFeature</Source>
      |         <SourceDirection>+X</SourceDirection>
      |         <FeatureName>+z surface</FeatureName>
      |       </SecondaryAxis>
      |     </Value>
      |   </Frame>
      | 
      |   <Frame>
      |     <Id>Frame2</Id>
      |     <Value>
      |       <Name>F2</Name>
      |       <Origin>
      |         <Source>GeometricFeature</Source>
      |         <FeatureName>+x surface</FeatureName>
      |       </Origin>
      |       <PrimaryAxis>
      |         <DefinedDirection>+Z</DefinedDirection>
      |         <Source>GeometricFeature</Source>
      |         <SourceDirection>+Z</SourceDirection>
      |         <FeatureName>+x surface</FeatureName>
      |       </PrimaryAxis>
      |       <SecondaryAxis>
      |         <DefinedDirection>+X</DefinedDirection>
      |         <Source>GeometricFeature</Source>
      |         <SourceDirection>+X</SourceDirection>
      |         <FeatureName>+z surface</FeatureName>
      |       </SecondaryAxis>
      |     </Value>
      |   </Frame>
      | 
      | </Frames>
  PS-Simulink Converter{,1..5} (6 alike) : nesl_utility/PS-Simulink Converter  PhysicalDomain=network_engine_domain  SubClassName=ps_output  LeftPortType=input  RightPortType=output  PseudoPeriodic=off  Frequencies=[]  VectorFormat=inherit  Unit=inherit  AffineConversion=off
  Simulink-PS Converter : nesl_utility/Simulink-PS Converter  PhysicalDomain=network_engine_domain  SubClassName=ps_input  LeftPortType=input  RightPortType=output  PseudoPeriodic=off  Frequencies=[]  NoiseDistribution=none  NoiseParameters=[]  Unit=1  AffineConversion=off  FilteringAndDerivatives=provide  SimscapeFilterOrder=1  InputFilterTimeConstant=0.001  UdotUserProvided=0
  Simulink-PS Converter1 : nesl_utility/Simulink-PS Converter  PhysicalDomain=network_engine_domain  SubClassName=ps_input  LeftPortType=input  RightPortType=output  PseudoPeriodic=off  Frequencies=[]  NoiseDistribution=none  NoiseParameters=[]  Unit=1  AffineConversion=off  FilteringAndDerivatives=provide  SimscapeFilterOrder=1  InputFilterTimeConstant=0.001  UdotUserProvided=0
  Spatial Contact Force : sm_lib/Forces and Torques/Spatial Contact Force  SenseSeparationDistance=off  NormalForceType=SmoothSpringDamper  NormalStiffness=contact_stiffness  NormalStiffnessUnits=N/m  NormalDamping=contact_damping  NormalDampingUnits=N/(m/s)  NormalTransitionRegionWidth=1e-4  NormalTransitionRegionWidthUnits=m  FrictionType=SmoothStickSlip  CoefficientOfStaticFriction=contact_static_friction  CoefficientOfDynamicFriction=contact_dynamic_friction  FrictionalCriticalVelocity=1e-2  FrictionalCriticalVelocityUnits=m/s  SenseContactSignal=off  SensePenetrationDepth=off  SenseNormalVelocity=off  SenseTangentialVelocity=off  SensingForceTorqueDirection=BaseOnFollower  SensingForceTorqueResolutionFrame=ContactFrame  SenseNormalForce=off  SenseNormalForceMagnitude=on  SenseNormalTorque=off  SenseFrictionalForce=off  SenseFrictionalForceMagnitude=on  SenseFrictionalTorque=off  SenseTotalForce=off  SenseTotalTorque=off  SenseContactBaseRotation=off  SenseContactBaseTranslation=off  SenseContactFollowerRotation=off  SenseContactFollowerTranslation=off  ZeroCrossDetectContactStartAndEnd=off
  Upper Leg : sm_lib/Body Elements/Brick Solid  BrickDimensions=upper_leg  BrickDimensionsUnits=m  ExportEntireGeometry=off  InertiaType=CalculateFromGeometry  BasedOnType=Density  Density=density  DensityUnits=kg/m^3  Mass=1  MassUnits=kg  CenterOfMass=[0 0 0]  CenterOfMassUnits=m  MomentsOfInertia=[1 1 1]  MomentsOfInertiaUnits=kg*m^2  ProductsOfInertia=[0 0 0]  ProductsOfInertiaUnits=kg*m^2  GraphicType=FromGeometry  MarkerShape=Sphere  MarkerSize=10  GraphicVisPropType=SimpleVisualProperties  GraphicDiffuseColor=robot_color  GraphicOpacity=1  GraphicSpecularColor=[0.5 0.5 0.5 1.0]  GraphicAmbientColor=[0.15 0.15 0.15 1.0]  GraphicEmissiveColor=[0.0 0.0 0.0 1.0]  GraphicShininess=75  DoExposeReferenceFrame=off  SerializedFrames=<Frames><Frame><Id>Frame1</Id><Value><Name>F1</Name><Origin><Source>GeometricFeature</Source><FeatureName>-x -y curve</FeatureName></Origin><PrimaryAxis><DefinedDirection>+Z</DefinedDirection><Source>GeometricFeature</Source><SourceDirection>+Z</SourceDirection><FeatureName>-y surface</FeatureName></PrimaryAxis><SecondaryAxis><DefinedDirection>+X</DefinedDirection><Source>GeometricFeature</Source><SourceDirection>+X</SourceDirection><FeatureName>+z surface</FeatureName></SecondaryAxis></Value></Frame><Frame><Id>Frame2</Id><Value><Name>F2</Name><Origin><Source>GeometricFeature</Source><FeatureName>+x -y curve</FeatureName></Origin><PrimaryAxis><DefinedDirection>+Z</DefinedDirection><Source>GeometricFeature</Source><SourceDirection>+Z</SourceDirection><FeatureName>-y surface</FeatureName></PrimaryAxis><SecondaryAxis><DefinedDirection>+X</DefinedDirection><Source>GeometricFeature</Source><SourceDirection>+X</SourceDirection><FeatureName>+z surface</FeatureName></SecondaryAxis></Value></Frame></Frames>
  B : PMIOPort  Side=Left
  G : PMIOPort  Port=2  Side=Right
  FL : Outport
  wires:
  PS-Simulink Converter/1 -> Bus Creator/6  "hip_speed"
  PS-Simulink Converter1/1 -> Bus Creator/5  "hip_angle"
  Demux/2 -> Simulink-PS Converter1/1
  Demux/1 -> Simulink-PS Converter/1
  torques/1 -> Demux/1
  PS-Simulink Converter3/1 -> Bus Creator/3  "knee_angle"
  PS-Simulink Converter2/1 -> Bus Creator/4  "knee_speed"
  PS-Simulink Converter4/1 -> Bus Creator/2  "force_magnitude"
  PS-Simulink Converter5/1 -> Bus Creator/1  "friction_force_magnitude"
  Bus Creator/1 -> FL/1
  connections:
  Spatial Contact Force/LConn1 -- G/RConn1
  Foot/RConn1 -- Leg to Foot/RConn1
  B/RConn1 -- Hip/LConn1
  Leg to Foot/LConn1 -- Lower Leg/RConn1
  Knee/RConn1 -- Lower Leg/LConn1
  Upper Leg/LConn1 -- Hip/RConn1
  Knee/LConn1 -- Upper Leg/RConn1
  Spatial Contact Force/RConn1 -- Foot/LConn1
  Simulink-PS Converter/RConn1 -- Hip/LConn2
  Hip/RConn2 -- PS-Simulink Converter1/LConn1
  Hip/RConn3 -- PS-Simulink Converter/LConn1
  Simulink-PS Converter1/RConn1 -- Knee/LConn2
  PS-Simulink Converter3/LConn1 -- Knee/RConn2
  PS-Simulink Converter2/LConn1 -- Knee/RConn3
  PS-Simulink Converter5/LConn1 -- Spatial Contact Force/RConn3
  PS-Simulink Converter4/LConn1 -- Spatial Contact Force/RConn2
